simulink model "dc_motor"  (R2024b)
settings: Solver=VariableStepAuto  StartTime=0.0  StopTime=10000  RelTol=1e-3
model workspace: external: MATLAB File C:\Users\PC\Documents\MATLAB\defined_params.m (data not in the file)
values from neighbouring files (symbols this model uses):
  b = 0.001    [defined_params.m]
  Jeq = 0.00010470588235294118    (= 0.000104705882353)    [defined_params.m]
  Kd = 2    [defined_params.m]
  Ke = 0.05    [defined_params.m]
  Kp = 40    [defined_params.m]
  Kt = 0.05    [defined_params.m]
  L = 0.005    [defined_params.m]
  N = 50    [defined_params.m]
  R = 2    [defined_params.m]
  target_rad = 4.0544924194335943    (= 4.05449241943)    [defined_params.m]
settings Model: DataDictionary=params.sldd  Creator=PC  LastModifiedBy=PC

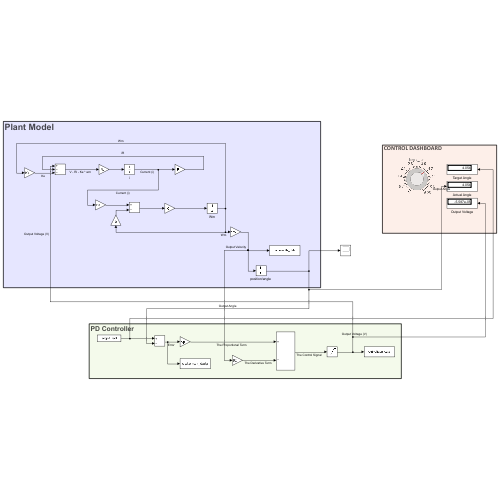
[thumbnail: Simulink's stored preview of the top-level diagram]
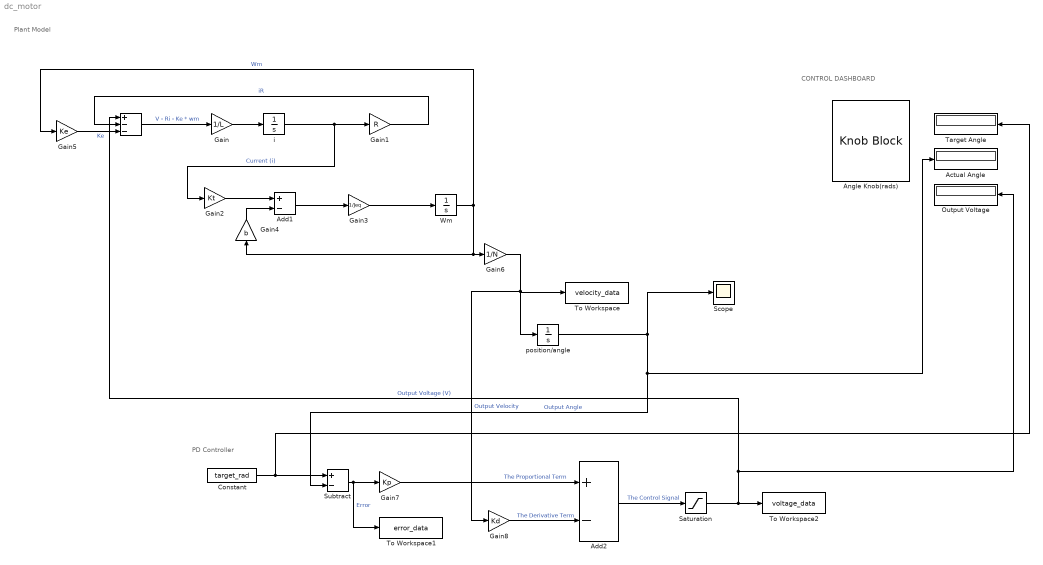
== system dc_motor ==
  note: PD Controller
  note: Plant Model
  note: CONTROL DASHBOARD
  " " : Sum  Inputs=+--
  Actual Angle : Display
  Add1 : Sum  Inputs=+-
  Add2 : Sum  Inputs=+-
  Angle Knob(rads) : KnobBlock  ScaleMax=6.28
  Constant : Constant  Value=target_rad
  Gain : Gain  Gain=1/L
  Gain1 : Gain  Gain=R
  Gain2 : Gain  Gain=Kt
  Gain3 : Gain  Gain=1/Jeq
  Gain4 : Gain  Gain=b
  Gain5 : Gain  Gain=Ke
  Gain6 : Gain  Gain=1/N
  Gain7 : Gain  Gain=Kp
  Gain8 : Gain  Gain=Kd
  Output Voltage : Display
  Saturation : Saturate  UpperLimit=12  LowerLimit=-12
  Scope : Scope
  Subtract : Sum  Inputs=+-
  Target Angle : Display
  To Workspace : ToWorkspace  VariableName=velocity_data  SampleTime=-1
  To Workspace1 : ToWorkspace  VariableName=error_data  SampleTime=-1
  To Workspace2 : ToWorkspace  VariableName=voltage_data  SampleTime=-1
  Wm : Integrator
  i : Integrator
  "position/angle " : Integrator
  wires:
  " "/1 -> Gain/1  "V - Ri - Ke * wm"
  Gain/1 -> i/1
  i/1 -> Gain1/1, Gain2/1  "Current (i)"
  Gain1/1 -> " "/2  "iR"
  Gain2/1 -> Add1/1
  Add1/1 -> Gain3/1
  Gain3/1 -> Wm/1
  Gain4/1 -> Add1/2
  Gain5/1 -> " "/3  "Ke"
  Wm/1 -> Gain6/1, Gain4/1, Gain5/1  "Wm"
  Gain6/1 -> Gain8/1, To Workspace/1, "position/angle "/1  "Output Velocity"
  Subtract/1 -> To Workspace1/1, Gain7/1  "Error"
  Gain7/1 -> Add2/1  "The Proportional Term"
  Gain8/1 -> Add2/2  "The Derivative Term"
  Add2/1 -> Saturation/1  "The Control Signal"
  "position/angle "/1 -> Actual Angle/1, Subtract/2, Scope/1  "Output Angle"
  Saturation/1 -> To Workspace2/1, Output Voltage/1, " "/1  "Output Voltage (V)"
  Constant/1 -> Subtract/1, Target Angle/1
